simulink model "PDplusController_iiwa"  (R2022b)
settings: Solver=ode4  StartTime=0.0  StopTime=T+5  FixedStep=0.001  RelTol=1e-3
values from neighbouring files (symbols this model uses):
  d = 10    [init_ImpedanceController.m]    (also in init_PDplusController.m)
  ddxd = dxd    [init_ImpedanceController.m]    (also in init_PDplusController.m)
  dq0 = ones(7,1)*pi/4    [init_ComputedTorque.m]    (also in init_ImpedanceController.m = zeros(7,1); init_PDplusController.m = zeros(7,1))
  dxd = zeros(size(xd))    [init_ImpedanceController.m]    (also in init_PDplusController.m)
  F_ext = -[0.9;0;-0.5;0;0;0]    [init_ImpedanceController.m]    (also in init_PDplusController.m)
  fall = 2    [init_ImpedanceController.m]    (also in init_PDplusController.m)
  k = 10    [init_ImpedanceController.m]    (also in init_PDplusController.m)
  l = 1    [init_ImpedanceController.m]
  q0 = [0; pi/4+0.5; 0; -pi/2; 0; pi/4+2;0]    [init_ComputedTorque.m]    (also in init_ImpedanceController.m = [0 pi/4 0 -pi/2 0 pi/4 0]'; init_PDplusController.m = [0 pi/4 0 -pi/2 0 pi/4 0]')
  T = 10    [init_ComputedTorque.m]    (also in init_ImpedanceController.m = 5; init_PDplusController.m = 5)
  x_T = [0.5 0.50 0.50 0 0 0]'    [init_ImpedanceController.m]    (also in init_PDplusController.m)
  xd = x_RPY_fromH(H)    [init_ImpedanceController.m]    (also in init_PDplusController.m)
undefined symbols (not defined in the file or in its folder): param_robot, X, Y, Z
libraries: sm_lib x66, nesl_utility x8
(part 2 of 2)

== system PDplusController_iiwa/Visualisierung/iiwa_link_ee ==
  Inertia : sm_lib/Body Elements/Inertia  InertiaType=Custom  Mass=0  MassUnits=kg  CenterOfMass=[0, 0, 0]  CenterOfMassUnits=m  MomentsOfInertia=[0, 0, 0]  MomentsOfInertiaUnits=kg*m^2  ProductsOfInertia=[0, 0, 0]  ProductsOfInertiaUnits=kg*m^2  GraphicType=None  MarkerShape=Inertia  MarkerSize=20  GraphicVisPropType=SimpleVisualProperties  GraphicDiffuseColor=[0.5 0.5 0.5]  GraphicSpecularColor=[0.5 0.5 0.5 1.0]  GraphicAmbientColor=[0.15 0.15 0.15 1.0]  GraphicEmissiveColor=[0.0 0.0 0.0 1.0]  GraphicShininess=75  GraphicOpacity=1.0
  InertiaOriginTransform : sm_lib/Frames and Transforms/Rigid Transform  TranslationMethod=Cartesian  TranslationStandardOffset=0  TranslationLengthUnit=m  TranslationStandardAxis=+Z  TranslationCartesianOffset=[0, 0, 0]  TranslationROffset=0  TranslationROffsetUnits=m  TranslationZOffset=0  TranslationZOffsetUnits=m  TranslationThetaOffset=0  TranslationThetaOffsetUnits=deg  RotationMethod=RotationSequence  RotationAngleUnits=deg  RotationStandardAxis=+Z  RotationAngle=0.0  RotationArbitraryAxis=[0 0 1]  FollAlignAxisA=+X  BaseAlignAxisA=+Y  FollAlignAxisB=+Y  BaseAlignAxisB=+Z  RotationSequenceAxes=BaseAxes  RotationSequence=XYZ  RotationSequenceAngles=[0, 0, 0]  RotationSequenceAnglesUnits=rad  RotationMatrix=[1 0 0; 0 1 0; 0 0 1]  Quaternion=[1 0 0 0]
  ReferenceFrame : sm_lib/Frames and Transforms/Reference Frame
  Visual : sm_lib/Body Elements/File Solid  ExtGeomFileName=./meshes/Stifthalterung.stl  UnitType=Custom  ExtGeomFileUnits=mm  StepReaderType=HEX  ExportConvexHullGeometry=off  InertiaType=Custom  Mass=0  MassUnits=kg  CenterOfMass=[0, 0, 0]  CenterOfMassUnits=m  MomentsOfInertia=[0, 0, 0]  MomentsOfInertiaUnits=kg*m^2  ProductsOfInertia=[0, 0, 0]  ProductsOfInertiaUnits=kg*m^2  BasedOnType=Density  Density=1000  DensityUnits=kg/m^3  DoExposeReferenceFrame=on  SerializedFrames=<Frames/>  GraphicType=FromGeometry  MarkerShape=Sphere  MarkerSize=10  GraphicVisPropType=SimpleVisualProperties  GraphicDiffuseColor=[0.4, 0.4, 0.4]  GraphicSpecularColor=[0.5 0.5 0.5 1.0]  GraphicAmbientColor=[0.15 0.15 0.15 1.0]  GraphicEmissiveColor=[0.0 0.0 0.0 1.0]  GraphicShininess=75  GraphicOpacity=1
  VisualOriginTransform : sm_lib/Frames and Transforms/Rigid Transform  TranslationMethod=Cartesian  TranslationStandardOffset=0  TranslationLengthUnit=m  TranslationStandardAxis=+Z  TranslationCartesianOffset=[0.025, 0, 0]  TranslationROffset=0  TranslationROffsetUnits=m  TranslationZOffset=0  TranslationZOffsetUnits=m  TranslationThetaOffset=0  TranslationThetaOffsetUnits=deg  RotationMethod=RotationSequence  RotationAngleUnits=deg  RotationStandardAxis=+Z  RotationAngle=0.0  RotationArbitraryAxis=[0 0 1]  FollAlignAxisA=+X  BaseAlignAxisA=+Y  FollAlignAxisB=+Y  BaseAlignAxisB=+Z  RotationSequenceAxes=BaseAxes  RotationSequence=XYZ  RotationSequenceAngles=[0, 0, 0]  RotationSequenceAnglesUnits=rad  RotationMatrix=[1 0 0; 0 1 0; 0 0 1]  Quaternion=[1 0 0 0]
  F : PMIOPort  Side=Left
  connections:
  F/RConn1 -- InertiaOriginTransform/LConn1 -- VisualOriginTransform/LConn1 -- ReferenceFrame/RConn1
  Inertia/RConn1 -- InertiaOriginTransform/RConn1
  Visual/RConn1 -- VisualOriginTransform/RConn1

== system PDplusController_iiwa/Visualisierung/world ==
  ReferenceFrame : sm_lib/Frames and Transforms/Reference Frame
  world_iiwa_joint_OriginTransform : sm_lib/Frames and Transforms/Rigid Transform  TranslationMethod=Cartesian  TranslationStandardOffset=0  TranslationLengthUnit=m  TranslationStandardAxis=+Z  TranslationCartesianOffset=param_robot.p_0  TranslationROffset=0  TranslationROffsetUnits=m  TranslationZOffset=0  TranslationZOffsetUnits=m  TranslationThetaOffset=0  TranslationThetaOffsetUnits=deg  RotationMethod=RotationMatrix  RotationAngleUnits=deg  RotationStandardAxis=+Z  RotationAngle=0.0  RotationArbitraryAxis=[0 0 1]  FollAlignAxisA=+X  BaseAlignAxisA=+Y  FollAlignAxisB=+Y  BaseAlignAxisB=+Z  RotationSequenceAxes=BaseAxes  RotationSequence=XYZ  RotationSequenceAngles=[0, 0, 0]  RotationSequenceAnglesUnits=rad  RotationMatrix=param_robot.R_0  Quaternion=[1 0 0 0]
  F : PMIOPort  Side=Left
  F1 : PMIOPort  Port=2  Side=Right
  connections:
  world_iiwa_joint_OriginTransform/RConn1 -- F1/RConn1
  ReferenceFrame/RConn1 -- F/RConn1 -- world_iiwa_joint_OriginTransform/LConn1

== matlab function PDplusController_iiwa/RobotDynamics/MATLAB Function ==
  data: q input; ddq output; dq input; tau input
function ddq  = fcn(q,dq,tau)
    [M, C, g, ~, ~, ~] = dynamics_iiwa(q,dq);
    ddq = M\(-C*dq - g + tau);
end

== matlab function PDplusController_iiwa/Subsystem/MATLAB Function ==
  data: q input; tau output; dq input; ddxd input; dxd input; xd input; F_ext input; q_0 input; tau_ext output; ex output; dex output; d input; k input
function [tau, tau_ext, ex,dex] = fcn(q, dq, ddxd, dxd, xd, F_ext, q_0,  d, k)

%Lambda_d = eye(6)*l;  % Gewichtsänderung
D_d= eye(6)*d; % Dämpfungsmatrix
K_d= eye(6)*k; % Steifigkeitsmatrix 
K_0= eye(7) * 1; 
K_q = eye(7) * 1;
dV_p =  K_q * (q-q_0); % Mit Hilfe von REGSYSI

[M, C, g, H, Jg, dJg] = dynamics_iiwa(q,dq);

x = x_RPY_fromH(H);
T = T_RPY(x);
J_a = T\Jg;
dx = J_a * dq; 
dT = dT_RPY(x,dx);
% J_g = T * J_a => inv(T)(dJ_g - dT *J_a) =  dJ_a 
dJ_a = T\(dJg - dT*J_a);
J_a_pseudo = M\(J_a') *inv(J_a*(M\(J_a'))) ;

dex = dx - dxd;
ex = x - xd;


Lambda = inv(J_a* (M\J_a'));
mu_ = Lambda*(J_a*(M\C)-dJ_a);
mu_x = mu_ * J_a_pseudo;
F_g = Lambda*J_a*(M\g);



%F = Lambda *ddxd + mu_ * dq + F_g - Lambda * inv(Lambda_d)*(D_d*dex + K_d*ex)+(eye(6)-Lambda*inv(Lambda_d))*F_ext;
F= Lambda * ddxd  +mu_*dq - mu_x *dex + F_g-D_d*dex-K_d*ex;

tau_n = (eye(7)-J_a'*J_a_pseudo') * (-K_0*dq - dV_p);
tau = J_a'*F + tau_n; % Über 7.46;
tau_ext = J_a'*F_ext;

== matlab function PDplusController_iiwa/Subsystem1/MATLAB Function1 ==
  data: t input; xd output; T input; x_0 input; x_T input; dxd output; ddxd output; xd_old input; dxd_old input; ddxd_old input
function [xd, dxd, ddxd] = fcn(t, T, x_0, x_T  , xd_old, dxd_old, ddxd_old)



if t < T

    a_3 = 10/T^3; 
    a_4 = -15/T^4; 
    a_5 = 6/T^5;
    
    s = a_3*t^3+a_4*t^4+a_5*t^5;
    ds = a_3*t^2*3 + 4 * a_4 * t^3 + 5*a_5*t^4;
    dds = 6*a_3*t + 12*a_4*t^2 + 20*a_5*t^3;
    
    xd = x_0 + s *(x_T-x_0);
    dxd = ds*(x_T-x_0);
    ddxd = dds*(x_T-x_0);

else
    xd = xd_old;
    dxd = dxd_old;
    ddxd = ddxd_old;
end

== matlab function PDplusController_iiwa/Subsystem1/MATLAB Function2 ==
  data: q input; tau output; dq input; ddxd input; dxd input; xd input; F_ext input; q_0 input; tau_ext output; ex output; dex output; d input; k input; m output
function [tau, tau_ext, ex,dex, m] = fcn(q, dq, ddxd, dxd, xd, F_ext, q_0,  d, k)

%Lambda_d = eye(6)*l;  % Gewichtsänderung
D_d= eye(6)*d; % Dämpfungsmatrix
K_d= eye(6)*k; % Steifigkeitsmatrix 
K_0= eye(7) * 1; 
K_q = eye(7) * 1;
dV_p =  K_q * (q-q_0); % Mit Hilfe von REGSYSI 

[M, C, g, H, Jg, dJg] = dynamics_iiwa(q,dq);

m = sqrt(det(Jg*Jg')); %4.62 (Manipulierbarkeit =0 -> Singlularität )  

x = x_RPY_fromH(H);
T = T_RPY(x);
J_a = T\Jg;
dx = J_a * dq; 
dT = dT_RPY(x,dx);
% J_g = T * J_a => inv(T)(dJ_g - dT *J_a) =  dJ_a 
dJ_a = T\(dJg - dT*J_a);
J_a_pseudo = M\(J_a') *inv(J_a*(M\(J_a'))) ;

dex = dx - dxd;
ex = x - xd;


Lambda = inv(J_a* (M\J_a'));
mu_ = Lambda*(J_a*(M\C)-dJ_a);
mu_x = mu_ * J_a_pseudo;
F_g = Lambda*J_a*(M\g);




F= Lambda * ddxd  +mu_*dq - mu_x *dex + F_g-D_d*dex-K_d*ex;

tau_n = (eye(7)-J_a'*J_a_pseudo') * (-K_0*dq - dV_p); % Nullraum Regelung
tau = J_a'*F + tau_n; % 7.42;
tau_ext = J_a'*F_ext;
